simulink model "dog_x_bit_true_2023a"  (R2024a)
settings: Solver=ode45  StartTime=0.0  StopTime=1.5*lsim*Ts  MaxStep=1/f0/2  RelTol=1e-6
values from neighbouring files (symbols this model uses):
  ft = (bint-1)*fbin    [exe_DOG_X_bit_true_2023a.m]    (also in exe_DOG_X_integer_true_two_paths_5b.m)
  g1 = g1_ideal*1    (= 4)    [exe_DOG_X_bit_true_2023a.m]    (also in exe_DOG_X_integer_true_two_paths_5b.m)
  Kvco = f0    (= 99840000)    [exe_DOG_X_bit_true_2023a.m]    (also in exe_DOG_X_integer_true_two_paths_5b.m)
  lvl = Vfs*10^(Input_signal_dB/20)    (= 0.242661009508)    [exe_DOG_X_bit_true_2023a.m]    (also in exe_DOG_X_integer_true_two_paths_5b.m = 0.125892541179)
  Nbsv1 = Nbvco+4    (= 9)    [exe_DOG_X_bit_true_2023a.m]    (also in exe_DOG_X_integer_true_two_paths_5b.m)
  Nbsv2 = Nbsv1+Nbext    [exe_DOG_X_bit_true_2023a.m]    (also in exe_DOG_X_integer_true_two_paths_5b.m)
  pnoi = 10^(-(60)/10)*(Vfs^2/2)    (= 5e-07)    [exe_DOG_X_bit_true_2023a.m]    (also in exe_DOG_X_integer_true_two_paths_5b.m)
  T2 = 1/f2    (= 4.06901041667e-08)    [exe_DOG_X_bit_true_2023a.m]    (also in exe_DOG_X_integer_true_two_paths_5b.m)
  Ts = 1/fs    (= 3.25520833333e-07)    [exe_DOG_X_bit_true_2023a.m]    (also in exe_DOG_X_integer_true_two_paths_5b.m)
  Vfs = 1    [exe_DOG_X_bit_true_2023a.m]    (also in exe_DOG_X_integer_true_two_paths_5b.m)
undefined symbols (not defined in the file or in its folder): fa, fb
libraries: simulink_extras x86, simulink x10
(part 4 of 4)

== system dog_x_bit_true_2023a/TOP/Subsystem/Noise_shaper_HSNR/first difference substraction (9 bit)/FA2 ==
  B0 : Inport
  B1 : Inport  Port=2
  Cin : Inport  Port=3
  Combinatorial Logic : CombinatorialLogic
  Demux : Demux  Outputs=2
  Mux : Mux  Inputs=3
  S : Outport
  Co : Outport  Port=2
  wires:
  Mux/1 -> Combinatorial Logic/1
  Combinatorial Logic/1 -> Demux/1
  B1/1 -> Mux/2
  Cin/1 -> Mux/3
  B0/1 -> Mux/1
  Demux/1 -> Co/1
  Demux/2 -> S/1

== system dog_x_bit_true_2023a/TOP/Subsystem/Noise_shaper_HSNR/first difference substraction (9 bit)/FA3 ==
  B0 : Inport
  B1 : Inport  Port=2
  Cin : Inport  Port=3
  Combinatorial Logic : CombinatorialLogic
  Demux : Demux  Outputs=2
  Mux : Mux  Inputs=3
  S : Outport
  Co : Outport  Port=2
  wires:
  Mux/1 -> Combinatorial Logic/1
  Combinatorial Logic/1 -> Demux/1
  B1/1 -> Mux/2
  Cin/1 -> Mux/3
  B0/1 -> Mux/1
  Demux/1 -> Co/1
  Demux/2 -> S/1

== system dog_x_bit_true_2023a/TOP/Subsystem/Noise_shaper_HSNR/first difference substraction (9 bit)/FA4 ==
  B0 : Inport
  B1 : Inport  Port=2
  Cin : Inport  Port=3
  Combinatorial Logic : CombinatorialLogic
  Demux : Demux  Outputs=2
  Mux : Mux  Inputs=3
  S : Outport
  Co : Outport  Port=2
  wires:
  Mux/1 -> Combinatorial Logic/1
  Combinatorial Logic/1 -> Demux/1
  B1/1 -> Mux/2
  Cin/1 -> Mux/3
  B0/1 -> Mux/1
  Demux/1 -> Co/1
  Demux/2 -> S/1

== system dog_x_bit_true_2023a/TOP/Subsystem/Noise_shaper_HSNR/first difference substraction (9 bit)/FA5 ==
  B0 : Inport
  B1 : Inport  Port=2
  Cin : Inport  Port=3
  Combinatorial Logic : CombinatorialLogic
  Demux : Demux  Outputs=2
  Mux : Mux  Inputs=3
  S : Outport
  Co : Outport  Port=2
  wires:
  Mux/1 -> Combinatorial Logic/1
  Combinatorial Logic/1 -> Demux/1
  B1/1 -> Mux/2
  Cin/1 -> Mux/3
  B0/1 -> Mux/1
  Demux/1 -> Co/1
  Demux/2 -> S/1

== system dog_x_bit_true_2023a/TOP/Subsystem/Noise_shaper_HSNR/first difference substraction (9 bit)/FA6 ==
  B0 : Inport
  B1 : Inport  Port=2
  Cin : Inport  Port=3
  Combinatorial Logic : CombinatorialLogic
  Demux : Demux  Outputs=2
  Mux : Mux  Inputs=3
  S : Outport
  Co : Outport  Port=2
  wires:
  Mux/1 -> Combinatorial Logic/1
  Combinatorial Logic/1 -> Demux/1
  B1/1 -> Mux/2
  Cin/1 -> Mux/3
  B0/1 -> Mux/1
  Demux/1 -> Co/1
  Demux/2 -> S/1

== system dog_x_bit_true_2023a/TOP/Subsystem/Noise_shaper_HSNR/first difference substraction (9 bit)/FA7 ==
  B0 : Inport
  B1 : Inport  Port=2
  Cin : Inport  Port=3
  Combinatorial Logic : CombinatorialLogic
  Demux : Demux  Outputs=2
  Mux : Mux  Inputs=3
  S : Outport
  Co : Outport  Port=2
  wires:
  Mux/1 -> Combinatorial Logic/1
  Combinatorial Logic/1 -> Demux/1
  B1/1 -> Mux/2
  Cin/1 -> Mux/3
  B0/1 -> Mux/1
  Demux/1 -> Co/1
  Demux/2 -> S/1

== system dog_x_bit_true_2023a/TOP/Subsystem/Noise_shaper_HSNR/first difference substraction (9 bit)/FA8 ==
  B0 : Inport
  B1 : Inport  Port=2
  Cin : Inport  Port=3
  Combinatorial Logic : CombinatorialLogic
  Demux : Demux  Outputs=2
  Mux : Mux  Inputs=3
  S : Outport
  Co : Outport  Port=2
  wires:
  Mux/1 -> Combinatorial Logic/1
  Combinatorial Logic/1 -> Demux/1
  B1/1 -> Mux/2
  Cin/1 -> Mux/3
  B0/1 -> Mux/1
  Demux/1 -> Co/1
  Demux/2 -> S/1

== system dog_x_bit_true_2023a/TOP/Subsystem/Noise_shaper_HSNR/first difference substraction (9 bit)2/FA ==
  B0 : Inport
  B1 : Inport  Port=2
  Cin : Inport  Port=3
  Combinatorial Logic : CombinatorialLogic
  Demux : Demux  Outputs=2
  Mux : Mux  Inputs=3
  S : Outport
  Co : Outport  Port=2
  wires:
  Mux/1 -> Combinatorial Logic/1
  Combinatorial Logic/1 -> Demux/1
  B1/1 -> Mux/2
  Cin/1 -> Mux/3
  B0/1 -> Mux/1
  Demux/1 -> Co/1
  Demux/2 -> S/1

== system dog_x_bit_true_2023a/TOP/Subsystem/Noise_shaper_HSNR/first difference substraction (9 bit)2/FA1 ==
  B0 : Inport
  B1 : Inport  Port=2
  Cin : Inport  Port=3
  Combinatorial Logic : CombinatorialLogic
  Demux : Demux  Outputs=2
  Mux : Mux  Inputs=3
  S : Outport
  Co : Outport  Port=2
  wires:
  Mux/1 -> Combinatorial Logic/1
  Combinatorial Logic/1 -> Demux/1
  B1/1 -> Mux/2
  Cin/1 -> Mux/3
  B0/1 -> Mux/1
  Demux/1 -> Co/1
  Demux/2 -> S/1

== system dog_x_bit_true_2023a/TOP/Subsystem/Noise_shaper_HSNR/first difference substraction (9 bit)2/FA2 ==
  B0 : Inport
  B1 : Inport  Port=2
  Cin : Inport  Port=3
  Combinatorial Logic : CombinatorialLogic
  Demux : Demux  Outputs=2
  Mux : Mux  Inputs=3
  S : Outport
  Co : Outport  Port=2
  wires:
  Mux/1 -> Combinatorial Logic/1
  Combinatorial Logic/1 -> Demux/1
  B1/1 -> Mux/2
  Cin/1 -> Mux/3
  B0/1 -> Mux/1
  Demux/1 -> Co/1
  Demux/2 -> S/1

== system dog_x_bit_true_2023a/TOP/Subsystem/Noise_shaper_HSNR/first difference substraction (9 bit)2/FA3 ==
  B0 : Inport
  B1 : Inport  Port=2
  Cin : Inport  Port=3
  Combinatorial Logic : CombinatorialLogic
  Demux : Demux  Outputs=2
  Mux : Mux  Inputs=3
  S : Outport
  Co : Outport  Port=2
  wires:
  Mux/1 -> Combinatorial Logic/1
  Combinatorial Logic/1 -> Demux/1
  B1/1 -> Mux/2
  Cin/1 -> Mux/3
  B0/1 -> Mux/1
  Demux/1 -> Co/1
  Demux/2 -> S/1

== system dog_x_bit_true_2023a/TOP/Subsystem/Noise_shaper_HSNR/first difference substraction (9 bit)2/FA4 ==
  B0 : Inport
  B1 : Inport  Port=2
  Cin : Inport  Port=3
  Combinatorial Logic : CombinatorialLogic
  Demux : Demux  Outputs=2
  Mux : Mux  Inputs=3
  S : Outport
  Co : Outport  Port=2
  wires:
  Mux/1 -> Combinatorial Logic/1
  Combinatorial Logic/1 -> Demux/1
  B1/1 -> Mux/2
  Cin/1 -> Mux/3
  B0/1 -> Mux/1
  Demux/1 -> Co/1
  Demux/2 -> S/1

== system dog_x_bit_true_2023a/TOP/Subsystem/Noise_shaper_HSNR/first difference substraction (9 bit)2/FA5 ==
  B0 : Inport
  B1 : Inport  Port=2
  Cin : Inport  Port=3
  Combinatorial Logic : CombinatorialLogic
  Demux : Demux  Outputs=2
  Mux : Mux  Inputs=3
  S : Outport
  Co : Outport  Port=2
  wires:
  Mux/1 -> Combinatorial Logic/1
  Combinatorial Logic/1 -> Demux/1
  B1/1 -> Mux/2
  Cin/1 -> Mux/3
  B0/1 -> Mux/1
  Demux/1 -> Co/1
  Demux/2 -> S/1

== system dog_x_bit_true_2023a/TOP/Subsystem/Noise_shaper_HSNR/first difference substraction (9 bit)2/FA6 ==
  B0 : Inport
  B1 : Inport  Port=2
  Cin : Inport  Port=3
  Combinatorial Logic : CombinatorialLogic
  Demux : Demux  Outputs=2
  Mux : Mux  Inputs=3
  S : Outport
  Co : Outport  Port=2
  wires:
  Mux/1 -> Combinatorial Logic/1
  Combinatorial Logic/1 -> Demux/1
  B1/1 -> Mux/2
  Cin/1 -> Mux/3
  B0/1 -> Mux/1
  Demux/1 -> Co/1
  Demux/2 -> S/1

== system dog_x_bit_true_2023a/TOP/Subsystem/Noise_shaper_HSNR/first difference substraction (9 bit)2/FA7 ==
  B0 : Inport
  B1 : Inport  Port=2
  Cin : Inport  Port=3
  Combinatorial Logic : CombinatorialLogic
  Demux : Demux  Outputs=2
  Mux : Mux  Inputs=3
  S : Outport
  Co : Outport  Port=2
  wires:
  Mux/1 -> Combinatorial Logic/1
  Combinatorial Logic/1 -> Demux/1
  B1/1 -> Mux/2
  Cin/1 -> Mux/3
  B0/1 -> Mux/1
  Demux/1 -> Co/1
  Demux/2 -> S/1

== system dog_x_bit_true_2023a/TOP/Subsystem/Noise_shaper_HSNR/first difference substraction (9 bit)2/FA8 ==
  B0 : Inport
  B1 : Inport  Port=2
  Cin : Inport  Port=3
  Combinatorial Logic : CombinatorialLogic
  Demux : Demux  Outputs=2
  Mux : Mux  Inputs=3
  S : Outport
  Co : Outport  Port=2
  wires:
  Mux/1 -> Combinatorial Logic/1
  Combinatorial Logic/1 -> Demux/1
  B1/1 -> Mux/2
  Cin/1 -> Mux/3
  B0/1 -> Mux/1
  Demux/1 -> Co/1
  Demux/2 -> S/1

== system dog_x_bit_true_2023a/TOP/Subsystem/Noise_shaper_HSNR/offset correction1/FA ==
  B0 : Inport
  B1 : Inport  Port=2
  Cin : Inport  Port=3
  Combinatorial Logic : CombinatorialLogic
  Demux : Demux  Outputs=2
  Mux : Mux  Inputs=3
  S : Outport
  Co : Outport  Port=2
  wires:
  Mux/1 -> Combinatorial Logic/1
  Combinatorial Logic/1 -> Demux/1
  B1/1 -> Mux/2
  Cin/1 -> Mux/3
  B0/1 -> Mux/1
  Demux/1 -> Co/1
  Demux/2 -> S/1

== system dog_x_bit_true_2023a/TOP/Subsystem/Noise_shaper_HSNR/offset correction1/FA1 ==
  B0 : Inport
  B1 : Inport  Port=2
  Cin : Inport  Port=3
  Combinatorial Logic : CombinatorialLogic
  Demux : Demux  Outputs=2
  Mux : Mux  Inputs=3
  S : Outport
  Co : Outport  Port=2
  wires:
  Mux/1 -> Combinatorial Logic/1
  Combinatorial Logic/1 -> Demux/1
  B1/1 -> Mux/2
  Cin/1 -> Mux/3
  B0/1 -> Mux/1
  Demux/1 -> Co/1
  Demux/2 -> S/1

== system dog_x_bit_true_2023a/TOP/Subsystem/Noise_shaper_HSNR/offset correction1/FA2 ==
  B0 : Inport
  B1 : Inport  Port=2
  Cin : Inport  Port=3
  Combinatorial Logic : CombinatorialLogic
  Demux : Demux  Outputs=2
  Mux : Mux  Inputs=3
  S : Outport
  Co : Outport  Port=2
  wires:
  Mux/1 -> Combinatorial Logic/1
  Combinatorial Logic/1 -> Demux/1
  B1/1 -> Mux/2
  Cin/1 -> Mux/3
  B0/1 -> Mux/1
  Demux/1 -> Co/1
  Demux/2 -> S/1

== system dog_x_bit_true_2023a/TOP/Subsystem/Noise_shaper_HSNR/offset correction1/FA3 ==
  B0 : Inport
  B1 : Inport  Port=2
  Cin : Inport  Port=3
  Combinatorial Logic : CombinatorialLogic
  Demux : Demux  Outputs=2
  Mux : Mux  Inputs=3
  S : Outport
  Co : Outport  Port=2
  wires:
  Mux/1 -> Combinatorial Logic/1
  Combinatorial Logic/1 -> Demux/1
  B1/1 -> Mux/2
  Cin/1 -> Mux/3
  B0/1 -> Mux/1
  Demux/1 -> Co/1
  Demux/2 -> S/1

== system dog_x_bit_true_2023a/TOP/Subsystem/Noise_shaper_HSNR/offset correction1/FA4 ==
  B0 : Inport
  B1 : Inport  Port=2
  Cin : Inport  Port=3
  Combinatorial Logic : CombinatorialLogic
  Demux : Demux  Outputs=2
  Mux : Mux  Inputs=3
  S : Outport
  Co : Outport  Port=2
  wires:
  Mux/1 -> Combinatorial Logic/1
  Combinatorial Logic/1 -> Demux/1
  B1/1 -> Mux/2
  Cin/1 -> Mux/3
  B0/1 -> Mux/1
  Demux/1 -> Co/1
  Demux/2 -> S/1

== system dog_x_bit_true_2023a/TOP/Subsystem/Noise_shaper_HSNR/offset correction1/FA5 ==
  B0 : Inport
  B1 : Inport  Port=2
  Cin : Inport  Port=3
  Combinatorial Logic : CombinatorialLogic
  Demux : Demux  Outputs=2
  Mux : Mux  Inputs=3
  S : Outport
  Co : Outport  Port=2
  wires:
  Mux/1 -> Combinatorial Logic/1
  Combinatorial Logic/1 -> Demux/1
  B1/1 -> Mux/2
  Cin/1 -> Mux/3
  B0/1 -> Mux/1
  Demux/1 -> Co/1
  Demux/2 -> S/1

== system dog_x_bit_true_2023a/TOP/Subsystem/Noise_shaper_HSNR/offset correction1/FA6 ==
  B0 : Inport
  B1 : Inport  Port=2
  Cin : Inport  Port=3
  Combinatorial Logic : CombinatorialLogic
  Demux : Demux  Outputs=2
  Mux : Mux  Inputs=3
  S : Outport
  Co : Outport  Port=2
  wires:
  Mux/1 -> Combinatorial Logic/1
  Combinatorial Logic/1 -> Demux/1
  B1/1 -> Mux/2
  Cin/1 -> Mux/3
  B0/1 -> Mux/1
  Demux/1 -> Co/1
  Demux/2 -> S/1

== system dog_x_bit_true_2023a/TOP/Subsystem/Noise_shaper_HSNR/offset correction1/FA7 ==
  B0 : Inport
  B1 : Inport  Port=2
  Cin : Inport  Port=3
  Combinatorial Logic : CombinatorialLogic
  Demux : Demux  Outputs=2
  Mux : Mux  Inputs=3
  S : Outport
  Co : Outport  Port=2
  wires:
  Mux/1 -> Combinatorial Logic/1
  Combinatorial Logic/1 -> Demux/1
  B1/1 -> Mux/2
  Cin/1 -> Mux/3
  B0/1 -> Mux/1
  Demux/1 -> Co/1
  Demux/2 -> S/1

== system dog_x_bit_true_2023a/TOP/Subsystem/Noise_shaper_HSNR/offset correction1/FA8 ==
  B0 : Inport
  B1 : Inport  Port=2
  Cin : Inport  Port=3
  Combinatorial Logic : CombinatorialLogic
  Demux : Demux  Outputs=2
  Mux : Mux  Inputs=3
  S : Outport
  Co : Outport  Port=2
  wires:
  Mux/1 -> Combinatorial Logic/1
  Combinatorial Logic/1 -> Demux/1
  B1/1 -> Mux/2
  Cin/1 -> Mux/3
  B0/1 -> Mux/1
  Demux/1 -> Co/1
  Demux/2 -> S/1

== system dog_x_bit_true_2023a/TOP/Subsystem/progressive_mux/Subsystem1/FA1 ==
  B0 : Inport
  B1 : Inport  Port=2
  Cin : Inport  Port=3
  Combinatorial Logic : CombinatorialLogic
  Demux : Demux  Outputs=2
  Mux : Mux  Inputs=3
  S : Outport
  Co : Outport  Port=2
  wires:
  Mux/1 -> Combinatorial Logic/1
  Combinatorial Logic/1 -> Demux/1
  B1/1 -> Mux/2
  Cin/1 -> Mux/3
  B0/1 -> Mux/1
  Demux/1 -> Co/1
  Demux/2 -> S/1

== system dog_x_bit_true_2023a/TOP/Subsystem/progressive_mux/Subsystem1/FA10 ==
  B0 : Inport
  B1 : Inport  Port=2
  Cin : Inport  Port=3
  Combinatorial Logic : CombinatorialLogic
  Demux : Demux  Outputs=2
  Mux : Mux  Inputs=3
  S : Outport
  Co : Outport  Port=2
  wires:
  Mux/1 -> Combinatorial Logic/1
  Combinatorial Logic/1 -> Demux/1
  B1/1 -> Mux/2
  Cin/1 -> Mux/3
  B0/1 -> Mux/1
  Demux/1 -> Co/1
  Demux/2 -> S/1

== system dog_x_bit_true_2023a/TOP/Subsystem/progressive_mux/Subsystem1/FA11 ==
  B0 : Inport
  B1 : Inport  Port=2
  Cin : Inport  Port=3
  Combinatorial Logic : CombinatorialLogic
  Demux : Demux  Outputs=2
  Mux : Mux  Inputs=3
  S : Outport
  Co : Outport  Port=2
  wires:
  Mux/1 -> Combinatorial Logic/1
  Combinatorial Logic/1 -> Demux/1
  B1/1 -> Mux/2
  Cin/1 -> Mux/3
  B0/1 -> Mux/1
  Demux/1 -> Co/1
  Demux/2 -> S/1

== system dog_x_bit_true_2023a/TOP/Subsystem/progressive_mux/Subsystem1/FA2 ==
  B0 : Inport
  B1 : Inport  Port=2
  Cin : Inport  Port=3
  Combinatorial Logic : CombinatorialLogic
  Demux : Demux  Outputs=2
  Mux : Mux  Inputs=3
  S : Outport
  Co : Outport  Port=2
  wires:
  Mux/1 -> Combinatorial Logic/1
  Combinatorial Logic/1 -> Demux/1
  B1/1 -> Mux/2
  Cin/1 -> Mux/3
  B0/1 -> Mux/1
  Demux/1 -> Co/1
  Demux/2 -> S/1

== system dog_x_bit_true_2023a/TOP/Subsystem/progressive_mux/Subsystem1/FA3 ==
  B0 : Inport
  B1 : Inport  Port=2
  Cin : Inport  Port=3
  Combinatorial Logic : CombinatorialLogic
  Demux : Demux  Outputs=2
  Mux : Mux  Inputs=3
  S : Outport
  Co : Outport  Port=2
  wires:
  Mux/1 -> Combinatorial Logic/1
  Combinatorial Logic/1 -> Demux/1
  B1/1 -> Mux/2
  Cin/1 -> Mux/3
  B0/1 -> Mux/1
  Demux/1 -> Co/1
  Demux/2 -> S/1

== system dog_x_bit_true_2023a/TOP/Subsystem/progressive_mux/Subsystem1/FA4 ==
  B0 : Inport
  B1 : Inport  Port=2
  Cin : Inport  Port=3
  Combinatorial Logic : CombinatorialLogic
  Demux : Demux  Outputs=2
  Mux : Mux  Inputs=3
  S : Outport
  Co : Outport  Port=2
  wires:
  Mux/1 -> Combinatorial Logic/1
  Combinatorial Logic/1 -> Demux/1
  B1/1 -> Mux/2
  Cin/1 -> Mux/3
  B0/1 -> Mux/1
  Demux/1 -> Co/1
  Demux/2 -> S/1

== system dog_x_bit_true_2023a/TOP/Subsystem/progressive_mux/Subsystem1/FA5 ==
  B0 : Inport
  B1 : Inport  Port=2
  Cin : Inport  Port=3
  Combinatorial Logic : CombinatorialLogic
  Demux : Demux  Outputs=2
  Mux : Mux  Inputs=3
  S : Outport
  Co : Outport  Port=2
  wires:
  Mux/1 -> Combinatorial Logic/1
  Combinatorial Logic/1 -> Demux/1
  B1/1 -> Mux/2
  Cin/1 -> Mux/3
  B0/1 -> Mux/1
  Demux/1 -> Co/1
  Demux/2 -> S/1

== system dog_x_bit_true_2023a/TOP/Subsystem/progressive_mux/Subsystem1/FA6 ==
  B0 : Inport
  B1 : Inport  Port=2
  Cin : Inport  Port=3
  Combinatorial Logic : CombinatorialLogic
  Demux : Demux  Outputs=2
  Mux : Mux  Inputs=3
  S : Outport
  Co : Outport  Port=2
  wires:
  Mux/1 -> Combinatorial Logic/1
  Combinatorial Logic/1 -> Demux/1
  B1/1 -> Mux/2
  Cin/1 -> Mux/3
  B0/1 -> Mux/1
  Demux/1 -> Co/1
  Demux/2 -> S/1

== system dog_x_bit_true_2023a/TOP/Subsystem/progressive_mux/Subsystem1/FA7 ==
  B0 : Inport
  B1 : Inport  Port=2
  Cin : Inport  Port=3
  Combinatorial Logic : CombinatorialLogic
  Demux : Demux  Outputs=2
  Mux : Mux  Inputs=3
  S : Outport
  Co : Outport  Port=2
  wires:
  Mux/1 -> Combinatorial Logic/1
  Combinatorial Logic/1 -> Demux/1
  B1/1 -> Mux/2
  Cin/1 -> Mux/3
  B0/1 -> Mux/1
  Demux/1 -> Co/1
  Demux/2 -> S/1

== system dog_x_bit_true_2023a/TOP/Subsystem/progressive_mux/Subsystem1/FA8 ==
  B0 : Inport
  B1 : Inport  Port=2
  Cin : Inport  Port=3
  Combinatorial Logic : CombinatorialLogic
  Demux : Demux  Outputs=2
  Mux : Mux  Inputs=3
  S : Outport
  Co : Outport  Port=2
  wires:
  Mux/1 -> Combinatorial Logic/1
  Combinatorial Logic/1 -> Demux/1
  B1/1 -> Mux/2
  Cin/1 -> Mux/3
  B0/1 -> Mux/1
  Demux/1 -> Co/1
  Demux/2 -> S/1

== system dog_x_bit_true_2023a/TOP/Subsystem/progressive_mux/Subsystem1/FA9 ==
  B0 : Inport
  B1 : Inport  Port=2
  Cin : Inport  Port=3
  Combinatorial Logic : CombinatorialLogic
  Demux : Demux  Outputs=2
  Mux : Mux  Inputs=3
  S : Outport
  Co : Outport  Port=2
  wires:
  Mux/1 -> Combinatorial Logic/1
  Combinatorial Logic/1 -> Demux/1
  B1/1 -> Mux/2
  Cin/1 -> Mux/3
  B0/1 -> Mux/1
  Demux/1 -> Co/1
  Demux/2 -> S/1

== system dog_x_bit_true_2023a/TOP/Subsystem/Noise_shaper_HDR/DCO/accumulator (11 bits)/FA1 ==
  B0 : Inport
  B1 : Inport  Port=2
  Cin : Inport  Port=3
  Combinatorial Logic : CombinatorialLogic
  Demux : Demux  Outputs=2
  Mux : Mux  Inputs=3
  S : Outport
  Co : Outport  Port=2
  wires:
  Demux/2 -> S/1
  Demux/1 -> Co/1
  B0/1 -> Mux/1
  Cin/1 -> Mux/3
  B1/1 -> Mux/2
  Combinatorial Logic/1 -> Demux/1
  Mux/1 -> Combinatorial Logic/1

== system dog_x_bit_true_2023a/TOP/Subsystem/Noise_shaper_HDR/DCO/accumulator (11 bits)/FA11 ==
  B0 : Inport
  B1 : Inport  Port=2
  Cin : Inport  Port=3
  Combinatorial Logic : CombinatorialLogic
  Demux : Demux  Outputs=2
  Mux : Mux  Inputs=3
  S : Outport
  Co : Outport  Port=2
  wires:
  Demux/2 -> S/1
  Demux/1 -> Co/1
  B0/1 -> Mux/1
  Cin/1 -> Mux/3
  B1/1 -> Mux/2
  Combinatorial Logic/1 -> Demux/1
  Mux/1 -> Combinatorial Logic/1

== system dog_x_bit_true_2023a/TOP/Subsystem/Noise_shaper_HDR/DCO/accumulator (11 bits)/FA12 ==
  B0 : Inport
  B1 : Inport  Port=2
  Cin : Inport  Port=3
  Combinatorial Logic : CombinatorialLogic
  Demux : Demux  Outputs=2
  Mux : Mux  Inputs=3
  S : Outport
  Co : Outport  Port=2
  wires:
  Demux/2 -> S/1
  Demux/1 -> Co/1
  B0/1 -> Mux/1
  Cin/1 -> Mux/3
  B1/1 -> Mux/2
  Combinatorial Logic/1 -> Demux/1
  Mux/1 -> Combinatorial Logic/1

== system dog_x_bit_true_2023a/TOP/Subsystem/Noise_shaper_HDR/DCO/accumulator (11 bits)/FA13 ==
  B0 : Inport
  B1 : Inport  Port=2
  Cin : Inport  Port=3
  Combinatorial Logic : CombinatorialLogic
  Demux : Demux  Outputs=2
  Mux : Mux  Inputs=3
  S : Outport
  Co : Outport  Port=2
  wires:
  Demux/2 -> S/1
  Demux/1 -> Co/1
  B0/1 -> Mux/1
  Cin/1 -> Mux/3
  B1/1 -> Mux/2
  Combinatorial Logic/1 -> Demux/1
  Mux/1 -> Combinatorial Logic/1

== system dog_x_bit_true_2023a/TOP/Subsystem/Noise_shaper_HDR/DCO/accumulator (11 bits)/FA2 ==
  B0 : Inport
  B1 : Inport  Port=2
  Cin : Inport  Port=3
  Combinatorial Logic : CombinatorialLogic
  Demux : Demux  Outputs=2
  Mux : Mux  Inputs=3
  S : Outport
  Co : Outport  Port=2
  wires:
  Demux/2 -> S/1
  Demux/1 -> Co/1
  B0/1 -> Mux/1
  Cin/1 -> Mux/3
  B1/1 -> Mux/2
  Combinatorial Logic/1 -> Demux/1
  Mux/1 -> Combinatorial Logic/1

== system dog_x_bit_true_2023a/TOP/Subsystem/Noise_shaper_HDR/DCO/accumulator (11 bits)/FA3 ==
  B0 : Inport
  B1 : Inport  Port=2
  Cin : Inport  Port=3
  Combinatorial Logic : CombinatorialLogic
  Demux : Demux  Outputs=2
  Mux : Mux  Inputs=3
  S : Outport
  Co : Outport  Port=2
  wires:
  Demux/2 -> S/1
  Demux/1 -> Co/1
  B0/1 -> Mux/1
  Cin/1 -> Mux/3
  B1/1 -> Mux/2
  Combinatorial Logic/1 -> Demux/1
  Mux/1 -> Combinatorial Logic/1

== system dog_x_bit_true_2023a/TOP/Subsystem/Noise_shaper_HDR/DCO/accumulator (11 bits)/FA4 ==
  B0 : Inport
  B1 : Inport  Port=2
  Cin : Inport  Port=3
  Combinatorial Logic : CombinatorialLogic
  Demux : Demux  Outputs=2
  Mux : Mux  Inputs=3
  S : Outport
  Co : Outport  Port=2
  wires:
  Demux/2 -> S/1
  Demux/1 -> Co/1
  B0/1 -> Mux/1
  Cin/1 -> Mux/3
  B1/1 -> Mux/2
  Combinatorial Logic/1 -> Demux/1
  Mux/1 -> Combinatorial Logic/1

== system dog_x_bit_true_2023a/TOP/Subsystem/Noise_shaper_HDR/DCO/accumulator (11 bits)/FA5 ==
  B0 : Inport
  B1 : Inport  Port=2
  Cin : Inport  Port=3
  Combinatorial Logic : CombinatorialLogic
  Demux : Demux  Outputs=2
  Mux : Mux  Inputs=3
  S : Outport
  Co : Outport  Port=2
  wires:
  Demux/2 -> S/1
  Demux/1 -> Co/1
  B0/1 -> Mux/1
  Cin/1 -> Mux/3
  B1/1 -> Mux/2
  Combinatorial Logic/1 -> Demux/1
  Mux/1 -> Combinatorial Logic/1

== system dog_x_bit_true_2023a/TOP/Subsystem/Noise_shaper_HDR/DCO/accumulator (11 bits)/FA6 ==
  B0 : Inport
  B1 : Inport  Port=2
  Cin : Inport  Port=3
  Combinatorial Logic : CombinatorialLogic
  Demux : Demux  Outputs=2
  Mux : Mux  Inputs=3
  S : Outport
  Co : Outport  Port=2
  wires:
  Demux/2 -> S/1
  Demux/1 -> Co/1
  B0/1 -> Mux/1
  Cin/1 -> Mux/3
  B1/1 -> Mux/2
  Combinatorial Logic/1 -> Demux/1
  Mux/1 -> Combinatorial Logic/1

== system dog_x_bit_true_2023a/TOP/Subsystem/Noise_shaper_HDR/DCO/accumulator (11 bits)/FA7 ==
  B0 : Inport
  B1 : Inport  Port=2
  Cin : Inport  Port=3
  Combinatorial Logic : CombinatorialLogic
  Demux : Demux  Outputs=2
  Mux : Mux  Inputs=3
  S : Outport
  Co : Outport  Port=2
  wires:
  Demux/2 -> S/1
  Demux/1 -> Co/1
  B0/1 -> Mux/1
  Cin/1 -> Mux/3
  B1/1 -> Mux/2
  Combinatorial Logic/1 -> Demux/1
  Mux/1 -> Combinatorial Logic/1

== system dog_x_bit_true_2023a/TOP/Subsystem/Noise_shaper_HDR/DCO/accumulator (11 bits)/FA8 ==
  B0 : Inport
  B1 : Inport  Port=2
  Cin : Inport  Port=3
  Combinatorial Logic : CombinatorialLogic
  Demux : Demux  Outputs=2
  Mux : Mux  Inputs=3
  S : Outport
  Co : Outport  Port=2
  wires:
  Demux/2 -> S/1
  Demux/1 -> Co/1
  B0/1 -> Mux/1
  Cin/1 -> Mux/3
  B1/1 -> Mux/2
  Combinatorial Logic/1 -> Demux/1
  Mux/1 -> Combinatorial Logic/1

== system dog_x_bit_true_2023a/TOP/Subsystem/Noise_shaper_HSNR/DCO/accumulator (11 bits)/FA1 ==
  B0 : Inport
  B1 : Inport  Port=2
  Cin : Inport  Port=3
  Combinatorial Logic : CombinatorialLogic
  Demux : Demux  Outputs=2
  Mux : Mux  Inputs=3
  S : Outport
  Co : Outport  Port=2
  wires:
  Demux/2 -> S/1
  Demux/1 -> Co/1
  B0/1 -> Mux/1
  Cin/1 -> Mux/3
  B1/1 -> Mux/2
  Combinatorial Logic/1 -> Demux/1
  Mux/1 -> Combinatorial Logic/1

== system dog_x_bit_true_2023a/TOP/Subsystem/Noise_shaper_HSNR/DCO/accumulator (11 bits)/FA11 ==
  B0 : Inport
  B1 : Inport  Port=2
  Cin : Inport  Port=3
  Combinatorial Logic : CombinatorialLogic
  Demux : Demux  Outputs=2
  Mux : Mux  Inputs=3
  S : Outport
  Co : Outport  Port=2
  wires:
  Demux/2 -> S/1
  Demux/1 -> Co/1
  B0/1 -> Mux/1
  Cin/1 -> Mux/3
  B1/1 -> Mux/2
  Combinatorial Logic/1 -> Demux/1
  Mux/1 -> Combinatorial Logic/1

== system dog_x_bit_true_2023a/TOP/Subsystem/Noise_shaper_HSNR/DCO/accumulator (11 bits)/FA12 ==
  B0 : Inport
  B1 : Inport  Port=2
  Cin : Inport  Port=3
  Combinatorial Logic : CombinatorialLogic
  Demux : Demux  Outputs=2
  Mux : Mux  Inputs=3
  S : Outport
  Co : Outport  Port=2
  wires:
  Demux/2 -> S/1
  Demux/1 -> Co/1
  B0/1 -> Mux/1
  Cin/1 -> Mux/3
  B1/1 -> Mux/2
  Combinatorial Logic/1 -> Demux/1
  Mux/1 -> Combinatorial Logic/1

== system dog_x_bit_true_2023a/TOP/Subsystem/Noise_shaper_HSNR/DCO/accumulator (11 bits)/FA13 ==
  B0 : Inport
  B1 : Inport  Port=2
  Cin : Inport  Port=3
  Combinatorial Logic : CombinatorialLogic
  Demux : Demux  Outputs=2
  Mux : Mux  Inputs=3
  S : Outport
  Co : Outport  Port=2
  wires:
  Demux/2 -> S/1
  Demux/1 -> Co/1
  B0/1 -> Mux/1
  Cin/1 -> Mux/3
  B1/1 -> Mux/2
  Combinatorial Logic/1 -> Demux/1
  Mux/1 -> Combinatorial Logic/1

== system dog_x_bit_true_2023a/TOP/Subsystem/Noise_shaper_HSNR/DCO/accumulator (11 bits)/FA2 ==
  B0 : Inport
  B1 : Inport  Port=2
  Cin : Inport  Port=3
  Combinatorial Logic : CombinatorialLogic
  Demux : Demux  Outputs=2
  Mux : Mux  Inputs=3
  S : Outport
  Co : Outport  Port=2
  wires:
  Demux/2 -> S/1
  Demux/1 -> Co/1
  B0/1 -> Mux/1
  Cin/1 -> Mux/3
  B1/1 -> Mux/2
  Combinatorial Logic/1 -> Demux/1
  Mux/1 -> Combinatorial Logic/1

== system dog_x_bit_true_2023a/TOP/Subsystem/Noise_shaper_HSNR/DCO/accumulator (11 bits)/FA3 ==
  B0 : Inport
  B1 : Inport  Port=2
  Cin : Inport  Port=3
  Combinatorial Logic : CombinatorialLogic
  Demux : Demux  Outputs=2
  Mux : Mux  Inputs=3
  S : Outport
  Co : Outport  Port=2
  wires:
  Demux/2 -> S/1
  Demux/1 -> Co/1
  B0/1 -> Mux/1
  Cin/1 -> Mux/3
  B1/1 -> Mux/2
  Combinatorial Logic/1 -> Demux/1
  Mux/1 -> Combinatorial Logic/1

== system dog_x_bit_true_2023a/TOP/Subsystem/Noise_shaper_HSNR/DCO/accumulator (11 bits)/FA4 ==
  B0 : Inport
  B1 : Inport  Port=2
  Cin : Inport  Port=3
  Combinatorial Logic : CombinatorialLogic
  Demux : Demux  Outputs=2
  Mux : Mux  Inputs=3
  S : Outport
  Co : Outport  Port=2
  wires:
  Demux/2 -> S/1
  Demux/1 -> Co/1
  B0/1 -> Mux/1
  Cin/1 -> Mux/3
  B1/1 -> Mux/2
  Combinatorial Logic/1 -> Demux/1
  Mux/1 -> Combinatorial Logic/1

== system dog_x_bit_true_2023a/TOP/Subsystem/Noise_shaper_HSNR/DCO/accumulator (11 bits)/FA5 ==
  B0 : Inport
  B1 : Inport  Port=2
  Cin : Inport  Port=3
  Combinatorial Logic : CombinatorialLogic
  Demux : Demux  Outputs=2
  Mux : Mux  Inputs=3
  S : Outport
  Co : Outport  Port=2
  wires:
  Demux/2 -> S/1
  Demux/1 -> Co/1
  B0/1 -> Mux/1
  Cin/1 -> Mux/3
  B1/1 -> Mux/2
  Combinatorial Logic/1 -> Demux/1
  Mux/1 -> Combinatorial Logic/1

== system dog_x_bit_true_2023a/TOP/Subsystem/Noise_shaper_HSNR/DCO/accumulator (11 bits)/FA6 ==
  B0 : Inport
  B1 : Inport  Port=2
  Cin : Inport  Port=3
  Combinatorial Logic : CombinatorialLogic
  Demux : Demux  Outputs=2
  Mux : Mux  Inputs=3
  S : Outport
  Co : Outport  Port=2
  wires:
  Demux/2 -> S/1
  Demux/1 -> Co/1
  B0/1 -> Mux/1
  Cin/1 -> Mux/3
  B1/1 -> Mux/2
  Combinatorial Logic/1 -> Demux/1
  Mux/1 -> Combinatorial Logic/1

== system dog_x_bit_true_2023a/TOP/Subsystem/Noise_shaper_HSNR/DCO/accumulator (11 bits)/FA7 ==
  B0 : Inport
  B1 : Inport  Port=2
  Cin : Inport  Port=3
  Combinatorial Logic : CombinatorialLogic
  Demux : Demux  Outputs=2
  Mux : Mux  Inputs=3
  S : Outport
  Co : Outport  Port=2
  wires:
  Demux/2 -> S/1
  Demux/1 -> Co/1
  B0/1 -> Mux/1
  Cin/1 -> Mux/3
  B1/1 -> Mux/2
  Combinatorial Logic/1 -> Demux/1
  Mux/1 -> Combinatorial Logic/1

== system dog_x_bit_true_2023a/TOP/Subsystem/Noise_shaper_HSNR/DCO/accumulator (11 bits)/FA8 ==
  B0 : Inport
  B1 : Inport  Port=2
  Cin : Inport  Port=3
  Combinatorial Logic : CombinatorialLogic
  Demux : Demux  Outputs=2
  Mux : Mux  Inputs=3
  S : Outport
  Co : Outport  Port=2
  wires:
  Demux/2 -> S/1
  Demux/1 -> Co/1
  B0/1 -> Mux/1
  Cin/1 -> Mux/3
  B1/1 -> Mux/2
  Combinatorial Logic/1 -> Demux/1
  Mux/1 -> Combinatorial Logic/1
